simulink model "model"  (R2022a)
settings: Solver=VariableStepAuto  StartTime=0.0  StopTime=20  RelTol=1e-3
values from neighbouring files (symbols this model uses):
  beta_r = deg2rad(beta)    [params.m]
  H = Fsl * rl + Fb * rz - Fsp * rp    [inertia.m]
  Jz = rl^2 * (1/3 * mbL + ml) + rp^2 * (1/3 * mbP + mp)    [inertia.m]
  rl = 0.235    [params.m]
  rw = 0.270    (= 0.27)    [params.m]
settings Model: Creator=Kamil  LastModifiedBy=Kamil

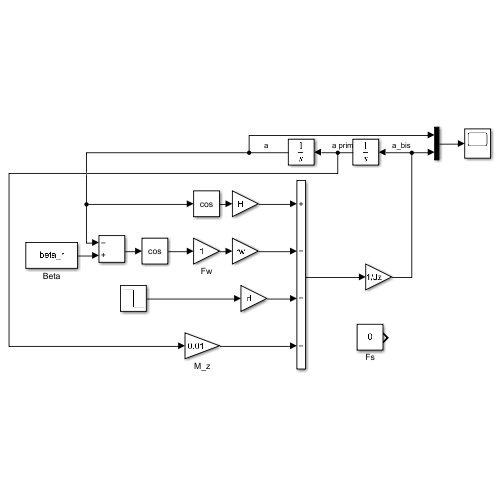
[thumbnail: Simulink's stored preview of the top-level diagram]
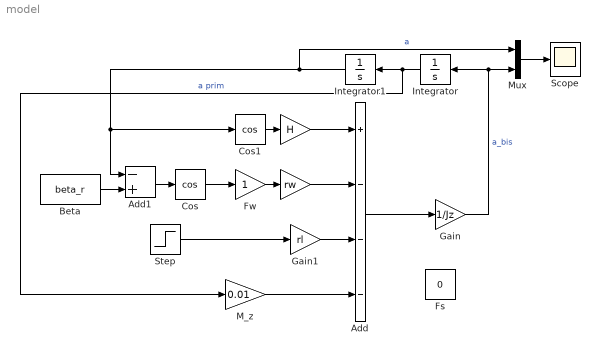
== system model ==
  " " : Gain  Gain=H
  "  " : Gain  Gain=rw
  Add : Sum  Inputs=+---
  Add1 : Sum  Inputs=-+
  Beta : Constant  Value=beta_r
  Cos : Trigonometry  Operator=cos
  Cos1 : Trigonometry  Operator=cos
  Fs : Constant  Value=0
  Fw : Gain
  Gain : Gain  Gain=1/Jz
  Gain1 : Gain  Gain=rl
  Integrator : Integrator
  Integrator1 : Integrator
  M_z : Gain  Gain=0.01
  Mux : Mux  Inputs=2
  Scope : Scope
  Step : Step  Time=0  After=-0.5  SampleTime=0
  wires:
  Integrator/1 -> M_z/1, Integrator1/1  "a prim"
  Integrator1/1 -> Mux/1, Add1/1, Cos1/1  "a"
  Step/1 -> Gain1/1
  Gain1/1 -> Add/3
  Fw/1 -> "  "/1
  Add1/1 -> Cos/1
  Beta/1 -> Add1/2
  Cos/1 -> Fw/1
  "  "/1 -> Add/2
  Cos1/1 -> " "/1
  " "/1 -> Add/1
  Add/1 -> Gain/1
  Gain/1 -> Mux/2, Integrator/1  "a_bis"
  Mux/1 -> Scope/1
  M_z/1 -> Add/4
